simulink model "az1"  (R2019b)
settings: Solver=FixedStepDiscrete  StartTime=0.0  StopTime=10.0  RelTol=1e-3
libraries: dspvision x2
settings Model: DataTypeOverride=Off  Creator=Mahyar Onsori  LastModifiedBy=Mahyar Onsori
settings DataIOCC: LimitDataPoints=on  SaveOutput=off  SaveTime=off
settings OptimizationCC: BlockReduction=off  ConditionallyExecuteInputs=off  DefaultParameterBehavior=Inlined  LifeSpan=inf
settings DebuggingCC: AlgebraicLoopMsg=error  SingleTaskRateTransMsg=error  AllowSymbolicDim=off  StrictBusMsg=ErrorOnBusTreatedAsVector  SFUnexpectedBacktrackingDiag=warning  SFNoUnconditionalDefaultTransitionDiag=warning  SFExecutionAtInitializationDiag=none  ArithmeticOperatorsInVariantConditions=warning
settings HardwareCC: ProdBitPerPointer=32  ProdBitPerSizeT=32  ProdBitPerPtrDiffT=32  ProdLargestAtomicFloat=None  ProdIntDivRoundTo=Undefined  ProdEndianess=Unspecified  ProdWordSize=32  ProdHWDeviceType=ASIC/FPGA->ASIC/FPGA  ProdEqTarget=off
settings SFSimCC: SimUseLocalCustomCode=off  CustomCodeUndefinedFunction=UseInterfaceOnly
settings RTWCC: RTWUseLocalCustomCode=off
settings CodeAppCC: StateflowObjectComments=on
settings GRTTargetCC: TargetLangStandard=C89/C90 (ANSI)  GeneratePreprocessorConditionals=Disable all
settings ConfigComp: CovScope=ReferencedModels  CovMetricSettings=dw  CovHtmlReporting=on  CovSaveCumulativeToWorkspaceVar=on  CovSaveSingleToWorkspaceVar=on  CovExternalEMLEnable=off  CovSFcnEnable=off

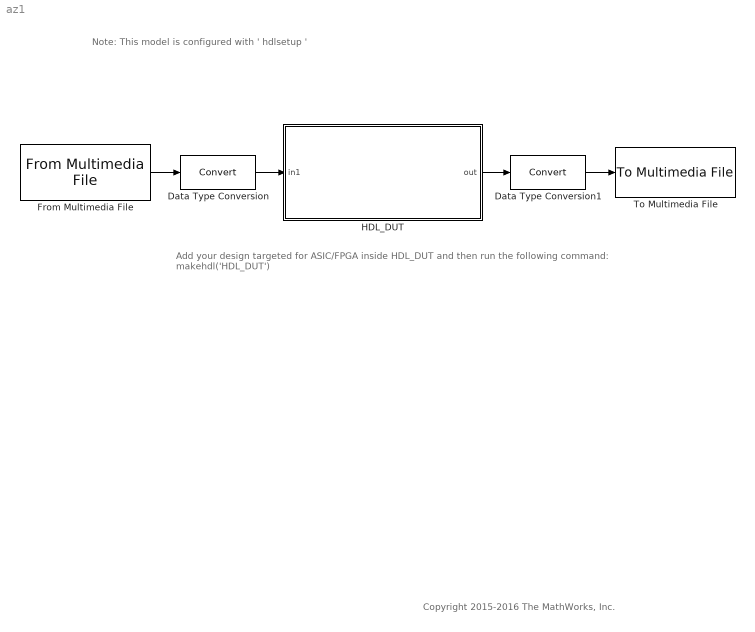
== system az1 ==
  note: Note: This model is configured with ' hdlsetup '
  note: Add your design targeted for ASIC/FPGA inside HDL_DUT and then run the following command:
      | makehdl('HDL_DUT')
  note: Copyright 2015-2016 The MathWorks, Inc.
  Data Type Conversion : DataTypeConversion  RndMeth=Nearest
  Data Type Conversion1 : DataTypeConversion
  From Multimedia File : dspvision/From Multimedia File  inputFilename=C:\Users\Mahyar Onsori\Desktop\FPGA1\hum.wav  readRange=[1 Inf]  loop=on  numPlays=1  outputStreams=Audio only  videoDataType=single  audioDataType=double  inheritSampleTime=on  userDefinedSampleTime=1/30  noAudioOutput=off  isIntensityVideo=off  fourcc=RGB  colorVideoFormat=Separate color signals  outputEOF=off  dataOrg=Column-major  audioFrameSize=1  computeAudioFrameSize=off  outSamplingMode=Sample based
      settings: SourceProductName=DSP System Toolbox  SourceProductBaseCode=DS
  HDL_DUT : Subsystem
  To Multimedia File : dspvision/To Multimedia File  outputFilename=C:\Users\Mahyar Onsori\Desktop\FPGA1\Result.wav  streamSelection=Audio only  videoCompressor=None (uncompressed)  audioCompressor=None (uncompressed)  imagePorts=Separate color signals  fileType=WAV  audioDatatype=16-bit integer  fourcc=RGB  videoQuality=75  mj2000CompFactor=10
      settings: SourceProductName=DSP System Toolbox  SourceProductBaseCode=DS
  wires:
  From Multimedia File/1 -> Data Type Conversion/1
  Data Type Conversion/1 -> HDL_DUT/1(in1)
  Data Type Conversion1/1 -> To Multimedia File/1
  HDL_DUT/1(out) -> Data Type Conversion1/1

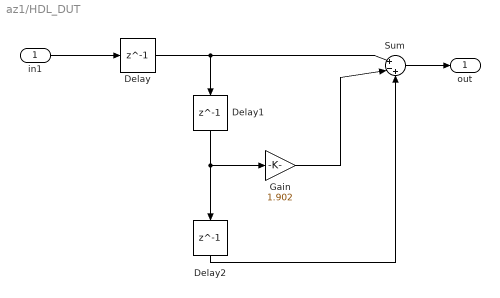
== system az1/HDL_DUT ==
  in1 : Inport  OutDataTypeStr=fixdt(1,16,14)
  Delay : Delay  DelayLength=1  InitialCondition=0
  Delay1 : Delay  DelayLength=1  InitialCondition=0
  Delay2 : Delay  DelayLength=1  InitialCondition=0
  Gain : Gain  Gain=1.902  OutDataTypeStr=fixdt(1,17,14)
  Sum : Sum  Inputs=|+-+  AccumDataTypeStr=fixdt(1,18,14)
  out : Outport  VectorParamsAs1DForOutWhenUnconnected=off
  wires:
  in1/1 -> Delay/1
  Delay/1 -> Delay1/1, Sum/1
  Delay1/1 -> Gain/1, Delay2/1
  Gain/1 -> Sum/2
  Delay2/1 -> Sum/3
  Sum/1 -> out/1
